simulink model "aconserversimulation"  (R2019b)
settings: Solver=FixedStepAuto  StartTime=0.0  StopTime=30  RelTol=1e-3
undefined symbols (not defined in the file or in its folder): Acid, Lead, sigbuilder_block
libraries: powerlib x39, simulink x14, powerlib_extras x9, electricdrivelib x3, re_lib x1
(part 1 of 2)
settings Model: Creator=28721  LastModifiedBy=conqu
settings SolverCC: ZeroCrossAlgorithm=Adaptive  AlgebraicLoopSolver=LineSearch
settings DataIOCC: ReturnWorkspaceOutputs=off
settings DebuggingCC: MaxConsecutiveZCsMsg=none  ArithmeticOperatorsInVariantConditions=warning
settings SFSimCC: SimUseLocalCustomCode=off  CustomCodeUndefinedFunction=UseInterfaceOnly
settings RTWCC: RTWUseLocalCustomCode=off

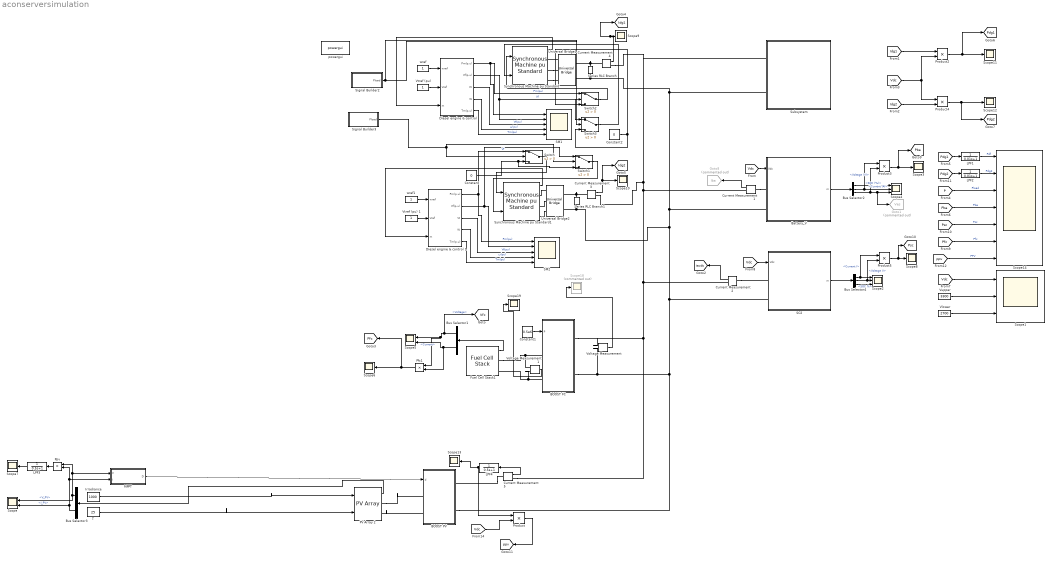
== system aconserversimulation ==
  BOOST FC : Subsystem
  BOOST PV : Subsystem
  Battery_V : Subsystem
      mask Display: image('D:\u盘文件\仿真\封装图片\timg (1).jpg');
  Bus Selector2 : BusSelector  OutputSignals=SOC (%),Current (A),Voltage (V)
  Bus Selector4 : BusSelector  OutputSignals=Current I,Voltage V,SOC %
  Bus Selector1 : BusSelector  OutputSignals=Voltage,Current
  Bus Selector3 : BusSelector  OutputSignals=V_PV,I_PV
  Constant : Constant  Value=0
  Constant1 : Constant  Value=0.5e6
  Constant2 : Constant  Value=0
  Current Measurement{1..5} (5 alike) : powerlib/Measurements/Current Measurement  PhasorSimulation=off  OutputType=Complex  PSBequivalent=0
      settings: SourceProductName=Simscape Electrical
  "Diesel engine & control " : Subsystem
  Diesel engine & control 1 : Subsystem
  Fuel Cell Stack1 : electricdrivelib/Extra Sources/Fuel Cell Stack  PresetModel=No (User-Defined)  FcType=Proton Exchange Membrane (PEM)  Detailed=Simplified  Eoc=[1600,1500]  NomVI=[800,2000]  EndVI=[1000,1800]  Nc=900  n=55  TOp=65  AirFr=2100  SuppPress=[1.5,1]  Comp=[99.95,21,1]  SignX=off  SignY=off  FlowRateH2=off  FlowRateAir=off  SystemTemp=off  SystemPH2=off  SystemPAir=off  FCDyn=on  FC_tau=1  Peak_O2=80  V_Under=10
      settings: SourceProductName=Simscape Electrical  SourceProductBaseCode=PS
  Goto1 : Goto  Commented=on  GotoTag=Ves  TagVisibility=global
  Goto8 : Goto  Commented=on  GotoTag=Iba  TagVisibility=global
  Irradiance : Constant  Value=1000
  LPF1 : TransferFcn  Denominator=[0.01 1]
  LPF2 : TransferFcn  Denominator=[0.01 1]
  LPF3 : TransferFcn  Denominator=[0.5 1]
  LPF4 : TransferFcn  Denominator=[0.5 1]
  MPPT : Subsystem
  PV Array 2 : re_lib/Solar/PV Array  Npar=100  Nser=55  PlotType=array @ 1000 W/m2 & specified temperatures  S_vec="[ 1000  500  100 ]"  Temp_C_vec="[ 50 25  ]"  ModuleName=Advanced Renewable Energy AREi-210W-M6-G  PlotWhenSelected=off  Pm=210.384  Ncell=60  Voc=36.3  Isc=7.74  Vm=29.22  Im=7.2  beta_Voc_pc=-0.35339  alpha_Isc_pc=0.055349  beta_Voc=-0.12828  alpha_Isc=0.004284  IL=7.7542  I0=2.0567e-10  nI=0.96787  Rsh=203.5777  Rs=0.37252  BAL=on  Tc=1e-6  Tfilter=5e-5
      link override Diode Rsh/Rsh_array_5%Sref: Value=Rsh_array5pc
      settings: SourceProductName=Simscape Electrical
  Pfc1 : Product
  Ppv : Product
  Product{,2..5} (5 alike) : Product
  SC2 : Subsystem
      mask Display: image('D:\u盘文件\仿真\封装图片\timg.jpg');
  SM1 : Scope  NumInputPorts=5
  SM2 : Scope  NumInputPorts=5
  Scope : Scope  NumInputPorts=2
  Scope1 : Scope  NumInputPorts=3
  Scope{3,6..13,19} (10 alike) : Scope
  Scope14 : Scope  NumInputPorts=7
  Scope18 : Scope  Commented=on
  Scope2 : Scope  NumInputPorts=3
  Scope4 : Scope  NumInputPorts=3
  Scope5 : Scope  NumInputPorts=2
  Series RLC Branch : powerlib/Elements/Series RLC Branch  LConnTagsString=__new0  RConnTagsString=__new0  BranchType=C  Resistance=1  Inductance=1e-3  SetiL0=off  InitialCurrent=0  Capacitance=1000e-6  Setx0=off  InitialVoltage=0  Measurements=None
      settings: SourceProductName=Simscape Electrical
  Series RLC Branch1 : powerlib/Elements/Series RLC Branch  LConnTagsString=__new0  RConnTagsString=__new0  BranchType=C  Resistance=1  Inductance=1e-3  SetiL0=off  InitialCurrent=0  Capacitance=1000e-6  Setx0=off  InitialVoltage=0  Measurements=None
      settings: SourceProductName=Simscape Electrical
  Signal Builder2 : Subsystem  Tag=STV Subsys  LoadFcn=sigbuilder_block('load');  StartFcn=sigbuilder_block('start');  StopFcn=sigbuilder_block('stop');  ClipboardFcn=sigbuilder_block('clipboard');  mask(Sigbuilder block){tuvar=[0:10]}
      mask help: Simulink:masks:SigbuilderBlock_MD
      mask init:
      | if ~strcmp(get_param(bdroot(gcbh),'SimulationStatus'),'stopped') tuvar = sigbuilder_block('maskInit'); end
      settings: CopyFcn=sigbuilder_block('copy');  DeleteFcn=sigbuilder_block('delete');  ModelCloseFcn=sigbuilder_block('modelClose');  PreSaveFcn=sigbuilder_block('preSave');  PauseFcn=sigbuilder_block('pause');  ContinueFcn=sigbuilder_block('continue');  NameChangeFcn=sigbuilder_block('namechange');  OpenFcn=sigbuilder_block('open',[381.6 135 550.8 400.2 ]);  CloseFcn=sigbuilder_block('close');
      mask Display: plot(0, 0, 100, 100,[2, 2, 32, 32, 2], [68, 8, 8, 68, 68],[32, 2], [38, 38], [32, 19, 2],[53, 60, 44], [32, 17, 17, 2],[16, 16, 31, 31]);txt = getActiveGroup(gcbh);text(2, 100, txt,'verticalAlignment', 'top');
  Signal Builder3 : Subsystem  Tag=STV Subsys  LoadFcn=sigbuilder_block('load');  StartFcn=sigbuilder_block('start');  StopFcn=sigbuilder_block('stop');  ClipboardFcn=sigbuilder_block('clipboard');  mask(Sigbuilder block){tuvar=[0:10]}
      mask help: Simulink:masks:SigbuilderBlock_MD
      mask init:
      | if ~strcmp(get_param(bdroot(gcbh),'SimulationStatus'),'stopped') tuvar = sigbuilder_block('maskInit'); end
      settings: CopyFcn=sigbuilder_block('copy');  DeleteFcn=sigbuilder_block('delete');  ModelCloseFcn=sigbuilder_block('modelClose');  PreSaveFcn=sigbuilder_block('preSave');  PauseFcn=sigbuilder_block('pause');  ContinueFcn=sigbuilder_block('continue');  NameChangeFcn=sigbuilder_block('namechange');  OpenFcn=sigbuilder_block('open',[381.6 135 550.8 400.2 ]);  CloseFcn=sigbuilder_block('close');
      mask Display: plot(0, 0, 100, 100,[2, 2, 32, 32, 2], [68, 8, 8, 68, 68],[32, 2], [38, 38], [32, 19, 2],[53, 60, 44], [32, 17, 17, 2],[16, 16, 31, 31]);txt = getActiveGroup(gcbh);text(2, 100, txt,'verticalAlignment', 'top');
  Subsystem : Subsystem
  Switch{,1..3} (4 alike) : Switch  Criteria=u2 > Threshold
  Synchronous Machine pu Standard : powerlib/Machines/Synchronous Machine pu Standard  PresetModel=No  MechanicalLoad=Mechanical power Pm  ShowDetailedParameters=on  RotorType=Salient-pole  Units=per unit standard parameters  MeasurementBus=off  NominalParameters="[3e6  2450 60]"  Reactances1=[ 1.81, 0.3, 0.23, 1.76, 0.65, 0.25, 0.15 ]  Reactances2=[ 1.56, 0.296, 0.177, 1.06, 0.177, 0.052 ]  dAxisTimeConstants=Short-circuit  qAxisTimeConstants=Open-circuit  TimeConstants1="[ 4.4849  0.0681  0.1  ]"  TimeConstants2=[ 8.0, 0.03, 1.0, 0.07 ]  TimeConstants3="[  4.49  0.0681  0.0513  ]"  TimeConstants4=[ 8.0, 0.03, 0.3371, 0.0295 ]  TimeConstants5=[ 3.7, 0.05, 0.05 ]  TimeConstants6=[ 1.3201, 0.023, 1.0, 0.07 ]  TimeConstants7=[ 3.7, 0.05, 0.05 ]  TimeConstants8=[ 1.3201, 0.0231, 0.3371, 0.0295 ]  StatorResistance=0.0036  Mechanical="[ 1.07  0 2]"  PolePairs=20  InitialConditions="[ 0  0  0  0  0  0  0  0  1 ]"  SetSaturation=on  Saturation=[0.6404,0.7127,0.8441,0.9214,0.9956,1.082,1.19,1.316,1.457;0.7,0.7698,0.8872,0.9466,0.9969,1.046,1.1,1.151,1.201]  LoadFlowParameters=[1,0,0,0,0]  TsPowergui=0  TsBlock=-1  IterativeModel=Trapezoidal non iterative  IterativeDiscreteModel=Trapezoidal non iterative  BusType=PV  Pref=0  Qref=0  Qmin=-inf  Qmax=inf  PLF=0  QLF=0
      settings: SourceProductName=Simscape Electrical
  Synchronous Machine pu Standard1 : powerlib/Machines/Synchronous Machine pu Standard  PresetModel=No  MechanicalLoad=Mechanical power Pm  ShowDetailedParameters=on  RotorType=Salient-pole  Units=per unit standard parameters  MeasurementBus=off  NominalParameters="[3e6  2450 60]"  Reactances1=[ 1.81, 0.3, 0.23, 1.76, 0.65, 0.25, 0.15 ]  Reactances2=[ 1.56, 0.296, 0.177, 1.06, 0.177, 0.052 ]  dAxisTimeConstants=Short-circuit  qAxisTimeConstants=Open-circuit  TimeConstants1="[ 4.4849  0.0681  0.1  ]"  TimeConstants2=[ 8.0, 0.03, 1.0, 0.07 ]  TimeConstants3="[  4.49  0.0681  0.0513  ]"  TimeConstants4=[ 8.0, 0.03, 0.3371, 0.0295 ]  TimeConstants5=[ 3.7, 0.05, 0.05 ]  TimeConstants6=[ 1.3201, 0.023, 1.0, 0.07 ]  TimeConstants7=[ 3.7, 0.05, 0.05 ]  TimeConstants8=[ 1.3201, 0.0231, 0.3371, 0.0295 ]  StatorResistance=0.0036  Mechanical="[ 1.07  0 2]"  PolePairs=20  InitialConditions="[ 0  0  0  0  0  0  0  0  1 ]"  SetSaturation=on  Saturation=[0.6404,0.7127,0.8441,0.9214,0.9956,1.082,1.19,1.316,1.457;0.7,0.7698,0.8872,0.9466,0.9969,1.046,1.1,1.151,1.201]  LoadFlowParameters=[1,0,0,0,0]  TsPowergui=0  TsBlock=-1  IterativeModel=Trapezoidal non iterative  IterativeDiscreteModel=Trapezoidal non iterative  BusType=PV  Pref=0  Qref=0  Qmin=-inf  Qmax=inf  PLF=0  QLF=0
      settings: SourceProductName=Simscape Electrical
  T : Constant  Value=25
  Universal Bridge1 : powerlib/Power Electronics/Universal Bridge  Arms=3  SnubberResistance=1e5  SnubberCapacitance=inf  Device=Diodes  Ron=1e-3  Lon=0  ForwardVoltages="[  0  0  ]"  ForwardVoltage=0  GTOparameters=[ 10e-6 , 20e-6 ]  IGBTparameters=[ 1e-6 , 2e-6 ]  Measurements=Device currents  Measurements_2=None  converterType=Rectifier
      settings: SourceProductName=Simscape Electrical
  Universal Bridge2 : powerlib/Power Electronics/Universal Bridge  Arms=3  SnubberResistance=1e5  SnubberCapacitance=inf  Device=Diodes  Ron=1e-3  Lon=0  ForwardVoltages="[  0  0  ]"  ForwardVoltage=0  GTOparameters=[ 10e-6 , 20e-6 ]  IGBTparameters=[ 1e-6 , 2e-6 ]  Measurements=Device currents  Measurements_2=None  converterType=Rectifier
      settings: SourceProductName=Simscape Electrical
  Vlower : Constant  Value=2700
  Voltage Measurement : powerlib/Measurements/Voltage Measurement  PhasorSimulation=off  OutputType=Complex  PSBequivalent=0
      settings: SourceProductName=Simscape Electrical
  Voltage Measurement1 : powerlib/Measurements/Voltage Measurement  PhasorSimulation=off  OutputType=Complex  PSBequivalent=0
      settings: SourceProductName=Simscape Electrical
  "Vtref (pu) " : Constant
  Vtref (pu) 1 : Constant
  Vupper : Constant  Value=3300
  powergui : powerlib/powergui  Priority=1  SimulationMode=Discrete  SampleTime=50e-6  frequency=60  Iterations=50  frequencyindice=0  Pbase=100e6  ErrMax=1e-4  UnitsV=kV  UnitsW=MW  buscounter=0  FunctionMessages=off  echomessages=off  EnableUseOfTLC=off  CurrentSourceSwitches=off  DisableSnubberDevices=off  DisableRonSwitches=off  DisableVfSwitches=off  DisplayEquations=off  AutomaticDiscreteSolvers=off  SolverType=Tustin/Backward Euler (TBE)  Interpol=off  ExternalGateDelay=off  methode=off  Ts=100  x0status=blocks  SPID=off  SwTol=0  HookPort=off  NonlinearTolerance=1e-4  nMaxIteration=100  ContinueOnMaxIteration=off  RestoreLinks=warning  ResistiveCurrentMeasurement=off  Frange=[0:2:500]  Ylog=off  Xlog=on  ShowGrid=off  save=off  variable=ZData  structure=Vdc  ZoomFFT=off  StartTime=0.0  cycles=1  DisplayStyle=1  fundamental=1  FreqAxis=off  MaxFrequency=1000  frequencyindicesteady=1  RmsSteady=1  display=off
      settings: SourceProductName=Simscape Electrical
  wref : Constant
  wref1 : Constant
  tag scope: Idg1=global, Idg2=global, Pba=global, Pdg1=global, Pdg2=global, Pfc=global, Psc=global, Vfc=global, iscdc=global, ppv=global
  wires:
  "Diesel engine & control "/4(W) -> SM1/4  "ω(pu)"
  "Diesel engine & control "/5(Tm(p.u)) -> SM1/5  "Tm(pu)"
  "Vtref (pu) "/1 -> "Diesel engine & control "/2(Vref)
  Synchronous Machine pu Standard/1 -> "Diesel engine & control "/3(m)
  "Diesel engine & control "/1(Pm(p.u)) -> Switch2/1, SM1/1  "Pm(pu)"
  "Diesel engine & control "/3(Vt) -> SM1/3  "Vt(pu)"
  "Diesel engine & control "/2(Vf(p.u)) -> Switch3/1, SM1/2  "Vf"
  wref/1 -> "Diesel engine & control "/1(wref)
  Bus Selector2/1 -> Scope4/1  "<SOC (%)>"
  Battery_V/1(m) -> Bus Selector2/1
  Bus Selector2/2 -> Product3/1, Scope4/2  "<Current (A)>"
  Bus Selector2/3 -> Product3/2, Goto1/1, Scope4/3  "<Voltage (V)>"
  Product3/1 -> [Pba], Scope3/1
  [Vdc] -> Battery_V/1(Vdc)
  Current Measurement4/1 -> [Idg1], Scope9/1
  [Idg1] -> Product2/1
  [Idg2] -> Product4/2
  [Vdc] -> Product2/2, Product4/1
  Product4/1 -> [Pdg2], Scope12/1
  Product2/1 -> Scope11/1, [Pdg1]
  Current Measurement1/1 -> Goto8/1
  LPF1/1 -> Scope14/1  "Pdf"
  LPF2/1 -> Scope14/2  "Pdg2"
  [P] -> Scope14/3  "Pload"
  wref1/1 -> Diesel engine & control 1/1(wref)
  Synchronous Machine pu Standard1/1 -> Diesel engine & control 1/3(m)
  Diesel engine & control 1/2(Vf(p.u)) -> Switch1/1, SM2/2  "Vf"
  Diesel engine & control 1/3(Vt) -> SM2/3  "Vt(pu)"
  Vtref (pu) 1/1 -> Diesel engine & control 1/2(Vref)
  Diesel engine & control 1/1(Pm(p.u)) -> Switch/1, SM2/1  "Pm(pu)"
  Diesel engine & control 1/5(Tm(p.u)) -> SM2/5  "Tm(pu)"
  Diesel engine & control 1/4(W) -> SM2/4  "ω(pu)"
  Current Measurement3/1 -> [Idg2], Scope10/1
  [Pba] -> Scope14/4  "Pba"
  [Vdc] -> Scope1/1
  Current Measurement2/1 -> [iscdc]
  Bus Selector4/3 -> Scope2/3  "<SOC %>"
  SC2/1(m) -> Bus Selector4/1
  [Vdc] -> SC2/1(Vdc)
  Bus Selector4/1 -> Product5/1, Scope2/1  "<Current I>"
  Product5/1 -> [Psc], Scope8/1
  Bus Selector4/2 -> Product5/2, Scope2/2  "<Voltage V>"
  [Psc] -> Scope14/5  "Psc"
  Constant1/1 -> BOOST FC/1(P)
  Bus Selector1/1 -> [Vfc], Pfc1/1, Scope5/1  "<Voltage>"
  Fuel Cell Stack1/1 -> Bus Selector1/1
  Pfc1/1 -> [Pfc], Scope6/1
  Bus Selector1/2 -> Pfc1/2, Scope5/2  "<Current>"
  [Pfc] -> Scope14/6  "Pfc"
  [Pdg2] -> LPF2/1
  [Pdg1] -> LPF1/1
  [ppv] -> Scope14/7  "PPV"
  Vupper/1 -> Scope1/2
  Vlower/1 -> Scope1/3
  Voltage Measurement/1 -> Scope18/1
  Voltage Measurement1/1 -> Scope19/1
  Constant/1 -> Switch1/3, Switch/3
  Switch/1 -> Synchronous Machine pu Standard1/1
  Switch1/1 -> Synchronous Machine pu Standard1/2
  Signal Builder3/1(Pload) -> Switch/2, Switch1/2
  Product/1 -> [ppv]
  [Vdc] -> Product/2
  Bus Selector3/2 -> Scope/2, Ppv/2, MPPT/2(I)  "<I_PV>"
  LPF4/1 -> Product/1, Scope13/1
  Irradiance/1 -> PV Array 2/1
  LPF3/1 -> Scope7/1
  Current Measurement5/1 -> LPF4/1
  MPPT/1(D) -> BOOST PV/1(d)
  Ppv/1 -> LPF3/1
  PV Array 2/1 -> Bus Selector3/1
  Bus Selector3/1 -> Scope/1, Ppv/1, MPPT/1(V)  "<V_PV>"
  T/1 -> PV Array 2/2
  Switch2/1 -> Synchronous Machine pu Standard/1
  Switch3/1 -> Synchronous Machine pu Standard/2
  Constant2/1 -> Switch2/3, Switch3/3
  Signal Builder2/1(Pload) -> Switch3/2, Switch2/2
  connections:
  Synchronous Machine pu Standard/RConn2 -- Universal Bridge1/LConn2
  Universal Bridge1/LConn1 -- Synchronous Machine pu Standard/RConn1
  Synchronous Machine pu Standard/RConn3 -- Universal Bridge1/LConn3
  Current Measurement1/LConn1 -- Battery_V/LConn1
  Voltage Measurement/LConn2 -- BOOST PV/RConn2 -- Series RLC Branch1/RConn1 -- Universal Bridge2/RConn2 -- Battery_V/LConn2 -- Series RLC Branch/RConn1 -- Universal Bridge1/RConn2 -- Subsystem/LConn2 -- SC2/LConn2 -- BOOST FC/RConn2
  Current Measurement2/RConn1 -- Current Measurement3/RConn1 -- Current Measurement4/RConn1 -- Subsystem/LConn1 -- Current Measurement1/RConn1 -- Current Measurement5/RConn1 -- Voltage Measurement/LConn1 -- BOOST FC/RConn1
  Current Measurement3/LConn1 -- Series RLC Branch1/LConn1 -- Universal Bridge2/RConn1
  Synchronous Machine pu Standard1/RConn2 -- Universal Bridge2/LConn2
  Universal Bridge2/LConn1 -- Synchronous Machine pu Standard1/RConn1
  Synchronous Machine pu Standard1/RConn3 -- Universal Bridge2/LConn3
  Current Measurement4/LConn1 -- Series RLC Branch/LConn1 -- Universal Bridge1/RConn1
  Current Measurement2/LConn1 -- SC2/LConn1
  BOOST FC/LConn2 -- Voltage Measurement1/LConn2 -- Fuel Cell Stack1/RConn2
  Fuel Cell Stack1/RConn1 -- Voltage Measurement1/LConn1 -- BOOST FC/LConn1
  Current Measurement5/LConn1 -- BOOST PV/RConn1
  PV Array 2/RConn1 -- BOOST PV/LConn1
  PV Array 2/RConn2 -- BOOST PV/LConn2

== system aconserversimulation/BOOST FC ==
  P : Inport
  Current Loop : Subsystem
  Current Measurement1 : powerlib/Measurements/Current Measurement  PhasorSimulation=off  OutputType=Complex  PSBequivalent=0
      settings: SourceProductName=Simscape Electrical
  Divide : Product  Inputs=*/
  Series RLC Branch7 : powerlib/Elements/Series RLC Branch  LConnTagsString=__new0  RConnTagsString=__new0  BranchType=C  Resistance=1  Inductance=1e-3  SetiL0=off  InitialCurrent=0  Capacitance=2000e-6  Setx0=off  InitialVoltage=0  Measurements=None
      settings: SourceProductName=Simscape Electrical
  boost converter : Subsystem
  Vdc+ : PMIOPort  Side=Right
  V+ : PMIOPort  Port=2  Side=Left
  Vdc- : PMIOPort  Port=3  Side=Right
  V- : PMIOPort  Port=4  Side=Left
  wires:
  Current Loop/1(d) -> boost converter/1(duty cycle)
  Current Measurement1/1 -> Current Loop/2(iLmes)
  Divide/1 -> Current Loop/1(iLref)
  P/1 -> Divide/1
  [Vfc] -> Divide/2
  connections:
  V+/RConn1 -- Current Measurement1/LConn1
  Current Measurement1/RConn1 -- boost converter/LConn1
  boost converter/LConn2 -- V-/RConn1
  boost converter/RConn1 -- Vdc+/RConn1 -- Series RLC Branch7/LConn1
  boost converter/RConn2 -- Vdc-/RConn1 -- Series RLC Branch7/RConn1

== system aconserversimulation/BOOST PV ==
  d : Inport
  Current Measurement2 : powerlib/Measurements/Current Measurement  PhasorSimulation=off  OutputType=Complex  PSBequivalent=0
      settings: SourceProductName=Simscape Electrical
  Current PI1 : Subsystem
  Scope4 : Scope
  boost converter : Subsystem
  Vdc+ : PMIOPort  Side=Right
  V+ : PMIOPort  Port=2  Side=Left
  Vdc- : PMIOPort  Port=3  Side=Right
  V- : PMIOPort  Port=4  Side=Left
  wires:
  d/1 -> Scope4/1, boost converter/1(duty cycle)
  connections:
  boost converter/RConn1 -- Vdc+/RConn1
  boost converter/LConn2 -- V-/RConn1
  boost converter/RConn2 -- Vdc-/RConn1
  boost converter/LConn1 -- V+/RConn1

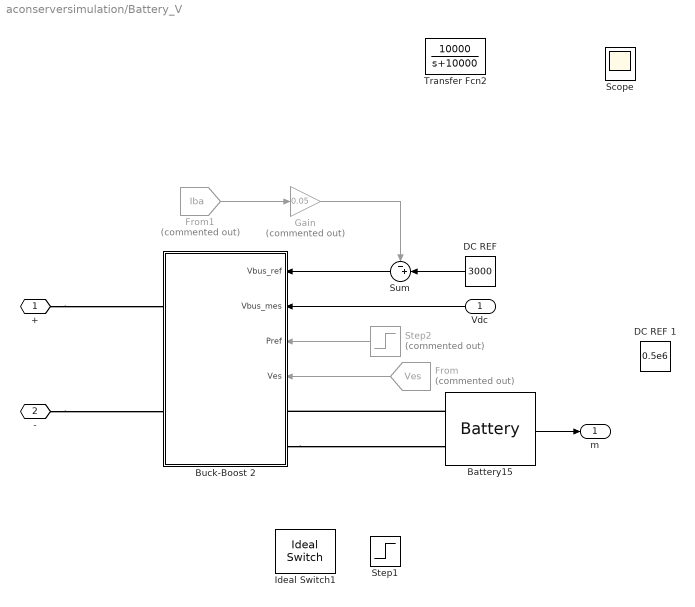
== system aconserversimulation/Battery_V ==
  Vdc : Inport
  Battery15 : electricdrivelib/Extra Sources/Battery  BatType=Lead-Acid  ShowTempParam=off  ThermalPreset=no  ShowAgeParam=off  NomV=2400  NomQ=100  SOC=40  Batt_Tr=30  PresetModel=on  MaxQ=104.1667  MinV=1800  FullV=2613.1579  Dis_rate=20  R=0.24  Normal_OP=31.0278  expZone="[2443.4211     0.33333333]"  current=[6.5 13 32.5]  Units=Time  Tci=20  NomT=20  T2=-30  MaxQ2=4.8  FullV2=7.1  Normal_OP2=5.655  expZone2="[6.58           1]"  Rca=0.6  ti=2000  Dp=0  Neq0=0  Tsim=1e6  Ta1=25  Qeol=5.4*0.9  Reol=0.013333*1.2  Char_age=[2.3478, 3]  Dis_age=[2.3478, 10]  N1=1500  N2=10500  N3=1000  N4=1400  Ta2=45  N5=950
      settings: SourceProductName=Simscape Electrical
  Buck-Boost 2 : Subsystem
  "DC REF " : Constant  Value=3000
  DC REF 1 : Constant  Value=0.5e6
  From : From  Commented=on  GotoTag=Ves  TagVisibility=global
  From1 : From  Commented=on  GotoTag=Iba  TagVisibility=global
  Gain : Gain  Commented=on  Gain=0.05
  Ideal Switch1 : powerlib/Power Electronics/Ideal Switch  Ron=0.001  Lon=0  IC=0  Rs=1e5  Cs=inf  Measurements=off
      settings: SourceProductName=Simscape Electrical
  Scope : Scope  NumInputPorts=2
  Step1 : Step  Time=2  SampleTime=0
  Step2 : Step  Commented=on  Time=3  Before=0.5e6  After=0.8e6  SampleTime=0
  Sum : Sum  Inputs=-+|
  Transfer Fcn2 : TransferFcn  Numerator=[10000]  Denominator=[1 10000]
  + : PMIOPort  Side=Left
  - : PMIOPort  Port=2  Side=Left
  m : Outport  VectorParamsAs1DForOutWhenUnconnected=off
  wires:
  Battery15/1 -> m/1
  Vdc/1 -> Buck-Boost 2/2(Vbus_mes)
  "DC REF "/1 -> Sum/2
  Sum/1 -> Buck-Boost 2/1(Vbus_ref)
  From1/1 -> Gain/1
  Gain/1 -> Sum/1
  From/1 -> Buck-Boost 2/4(Ves)
  Step2/1 -> Buck-Boost 2/3(Pref)
  connections:
  -/RConn1 -- Buck-Boost 2/RConn2
  Buck-Boost 2/LConn2 -- Battery15/LConn2
  +/RConn1 -- Buck-Boost 2/RConn1
  Battery15/LConn1 -- Buck-Boost 2/LConn1

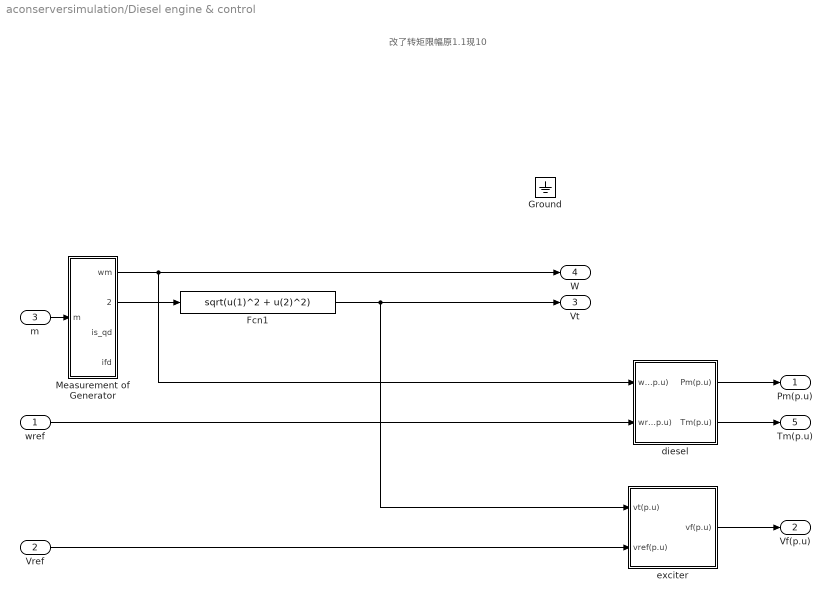
== system aconserversimulation/Diesel engine & control  ==
  note: 改了转矩限幅原1.1现10
  wref : Inport
  Vref : Inport  Port=2
  m : Inport  Port=3
  Fcn1 : Fcn  Expr=sqrt(u(1)^2 + u(2)^2)
  Ground : Ground
  Measurement of Generator : Subsystem
  diesel : Subsystem
  exciter : Subsystem
  Pm(p.u) : Outport  VectorParamsAs1DForOutWhenUnconnected=off
  Vf(p.u) : Outport  Port=2  VectorParamsAs1DForOutWhenUnconnected=off
  Vt : Outport  Port=3  VectorParamsAs1DForOutWhenUnconnected=off
  W : Outport  Port=4  VectorParamsAs1DForOutWhenUnconnected=off
  Tm(p.u) : Outport  Port=5  VectorParamsAs1DForOutWhenUnconnected=off
  wires:
  m/1 -> Measurement of Generator/1(m)
  Measurement of Generator/2(vs_qd) -> Fcn1/1
  Fcn1/1 -> exciter/1(vt(p.u)), Vt/1
  Measurement of Generator/1(wm) -> diesel/1(wm(p.u)), W/1
  wref/1 -> diesel/2(wref(p.u))
  diesel/2(Tm(p.u)) -> Tm(p.u)/1
  diesel/1(Pm(p.u)) -> Pm(p.u)/1
  Vref/1 -> exciter/2(vref(p.u))
  exciter/1(vf(p.u)) -> Vf(p.u)/1

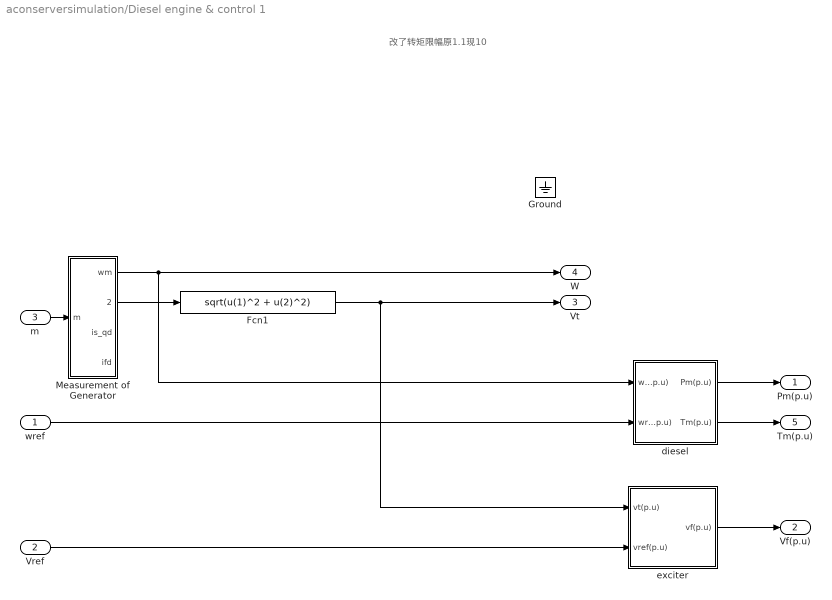
== system aconserversimulation/Diesel engine & control 1 ==
  note: 改了转矩限幅原1.1现10
  wref : Inport
  Vref : Inport  Port=2
  m : Inport  Port=3
  Fcn1 : Fcn  Expr=sqrt(u(1)^2 + u(2)^2)
  Ground : Ground
  Measurement of Generator : Subsystem
  diesel : Subsystem
  exciter : Subsystem
  Pm(p.u) : Outport  VectorParamsAs1DForOutWhenUnconnected=off
  Vf(p.u) : Outport  Port=2  VectorParamsAs1DForOutWhenUnconnected=off
  Vt : Outport  Port=3  VectorParamsAs1DForOutWhenUnconnected=off
  W : Outport  Port=4  VectorParamsAs1DForOutWhenUnconnected=off
  Tm(p.u) : Outport  Port=5  VectorParamsAs1DForOutWhenUnconnected=off
  wires:
  m/1 -> Measurement of Generator/1(m)
  Measurement of Generator/2(vs_qd) -> Fcn1/1
  Fcn1/1 -> exciter/1(vt(p.u)), Vt/1
  Measurement of Generator/1(wm) -> diesel/1(wm(p.u)), W/1
  wref/1 -> diesel/2(wref(p.u))
  diesel/2(Tm(p.u)) -> Tm(p.u)/1
  diesel/1(Pm(p.u)) -> Pm(p.u)/1
  Vref/1 -> exciter/2(vref(p.u))
  exciter/1(vf(p.u)) -> Vf(p.u)/1

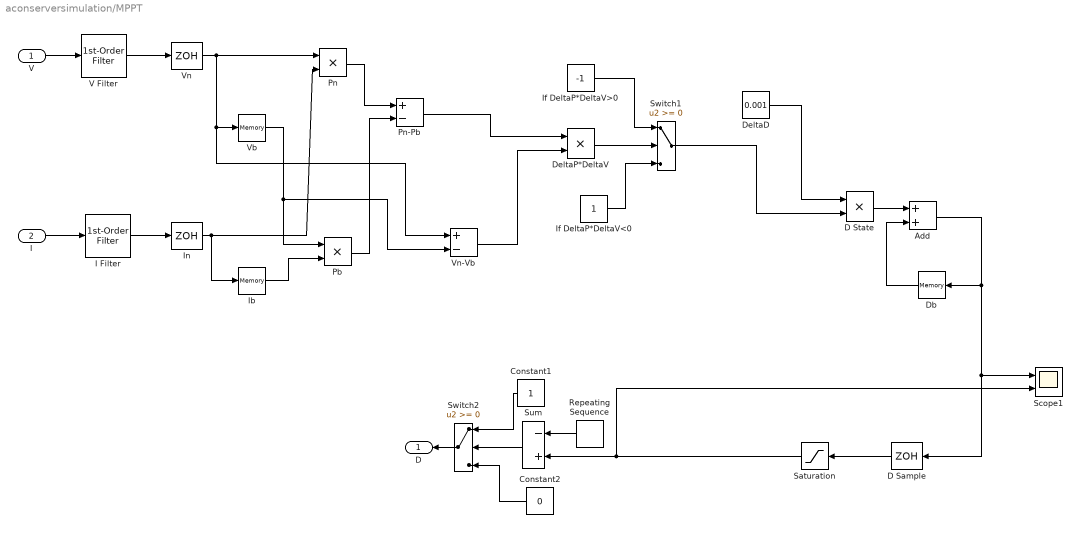
== system aconserversimulation/MPPT ==
  V : Inport
  I : Inport  Port=2
  Add : Sum
  Constant1 : Constant  SampleTime=-1
  Constant2 : Constant  Value=0  SampleTime=-1
  D Sample : ZeroOrderHold  SampleTime=1e-4
  D State : Product  RndMeth=Zero
  Db : Memory  InheritSampleTime=on  LinearizeAsDelay=on
  DeltaD : Constant  Value=0.001
  DeltaP*DeltaV : Product  RndMeth=Zero
  I Filter : powerlib_extras/Control  Blocks/1st-Order  Filter  FilterType=Lowpass  Tc=1e-3  Initialize=off  Vac_Init=[0.8 -25 60]  Vdc_Init=-0.4  PlotResponse=off  param1=[1 500 1]
      settings: SourceProductName=Simscape Electrical  SourceProductBaseCode=PS
  Ib : Memory  InheritSampleTime=on  LinearizeAsDelay=on
  If DeltaP*DeltaV<0 : Constant
  If DeltaP*DeltaV>0 : Constant  Value=-1
  In : ZeroOrderHold  SampleTime=1e-4
  Pb : Product  RndMeth=Zero
  Pn : Product  RndMeth=Zero
  Pn-Pb : Sum  Inputs=+-
  Repeating Sequence : simulink/Sources/Repeating Sequence  rep_seq_t=[0 3.9e-3 4e-3]  rep_seq_y=[0 1 0]
  Saturation : Saturate  UpperLimit=0.8  LowerLimit=0
  Scope1 : Scope  NumInputPorts=2
  Sum : Sum  Inputs=-+  SaturateOnIntegerOverflow=on
  Switch1 : Switch
  Switch2 : Switch
  V Filter : powerlib_extras/Control  Blocks/1st-Order  Filter  FilterType=Lowpass  Tc=1e-3  Initialize=off  Vac_Init=[0.8 -25 60]  Vdc_Init=-0.4  PlotResponse=off  param1=[1 500 1]
      settings: SourceProductName=Simscape Electrical  SourceProductBaseCode=PS
  Vb : Memory  InheritSampleTime=on  LinearizeAsDelay=on
  Vn : ZeroOrderHold  SampleTime=1e-4
  Vn-Vb : Sum  Inputs=+-
  D : Outport  VectorParamsAs1DForOutWhenUnconnected=off
  wires:
  V/1 -> V Filter/1
  I/1 -> I Filter/1
  V Filter/1 -> Vn/1
  I Filter/1 -> In/1
  In/1 -> Ib/1, Pn/2
  Vn/1 -> Pn/1, Vb/1, Vn-Vb/1
  Ib/1 -> Pb/2
  Vb/1 -> Pb/1, Vn-Vb/2
  Pn/1 -> Pn-Pb/1
  Pb/1 -> Pn-Pb/2
  D State/1 -> Add/1
  Constant2/1 -> Switch2/3
  Constant1/1 -> Switch2/1
  Sum/1 -> Switch2/2
  Repeating Sequence/1 -> Sum/1
  Add/1 -> Db/1, D Sample/1, Scope1/1
  Switch2/1 -> D/1
  Db/1 -> Add/2
  D Sample/1 -> Saturation/1
  Pn-Pb/1 -> DeltaP*DeltaV/1
  Vn-Vb/1 -> DeltaP*DeltaV/2
  DeltaP*DeltaV/1 -> Switch1/2
  If DeltaP*DeltaV>0/1 -> Switch1/1
  If DeltaP*DeltaV<0/1 -> Switch1/3
  Switch1/1 -> D State/2
  DeltaD/1 -> D State/1
  Saturation/1 -> Sum/2, Scope1/2

== system aconserversimulation/SC2 ==
  Vdc : Inport
  "Buck-Boost 1 " : Subsystem
  DC REF 1 : Constant  Value=3000
  Gain : Gain  Gain=0.1
  Sum : Sum  Inputs=-+|
  Supercapacitor : electricdrivelib/Extra Sources/Supercapacitor  C=2200  Rdc=8.9e-3  Voltage=1500  Ns=18  Np=1  Vinit=1200  Temp=25  PresetModel=off  EstParam=off  Nc=1  r=1e-9  epsilon=6.0208e-10  Ich=10  Vstern="[0.161  2.7  7.8]"  Self_dis=on  Ioc=10  Vself="[48  47.8  47.06  44.65]"  demandeplot=off  I="[10  20 100  500]"  Units=sec  Vmax=0  If=0  deltaV=0  alpha=0  sec=0
      settings: SourceProductName=Simscape Electrical  SourceProductBaseCode=PS
  Transfer Fcn2 : TransferFcn  Numerator=[1 0]  Denominator=[1 1000]
  + : PMIOPort  Side=Left
  - : PMIOPort  Port=2  Side=Left
  m : Outport  VectorParamsAs1DForOutWhenUnconnected=off
  wires:
  Supercapacitor/1 -> m/1
  Vdc/1 -> "Buck-Boost 1 "/2(Vbus_mes)
  [iscdc] -> Gain/1
  DC REF 1/1 -> Sum/2
  Sum/1 -> "Buck-Boost 1 "/1(Vbus_ref)
  connections:
  Supercapacitor/LConn1 -- "Buck-Boost 1 "/LConn1
  Supercapacitor/LConn2 -- "Buck-Boost 1 "/LConn2
  "Buck-Boost 1 "/RConn1 -- +/RConn1
  "Buck-Boost 1 "/RConn2 -- -/RConn1

== system aconserversimulation/Signal Builder2 ==
  Demux : Demux  Tag=STV Demux  Outputs=1
  FromWs : FromWorkspace  Tag=STV FromWs  VariableName=tuvar  SampleTime=0
      SigBuilderData=|
      | common.afterFinalStr = 'Extrapolate'
      | common.sampleTime = 0
      | dataSet.timeRange = [0 20]
      | dataSet.name = 'Group 1'
      | sbobj.Groups.Name = 'Group 1'
      | sbobj.Groups.Signals.Name = 'Pload'
      | sbobj.Groups.Signals.XData = [0 4 10 10 12 16 20]
      | sbobj.Groups.Signals.YData = [0 0 0 1 1 1 1]
      | sbobj.Groups.TimeRange = [0 20]
  Pload : Outport  Tag=STV Outport  VectorParamsAs1DForOutWhenUnconnected=off
  wires:
  FromWs/1 -> Demux/1
  Demux/1 -> Pload/1

== system aconserversimulation/Signal Builder3 ==
  Demux : Demux  Tag=STV Demux  Outputs=1
  FromWs : FromWorkspace  Tag=STV FromWs  VariableName=tuvar  SampleTime=0
      SigBuilderData=|
      | common.afterFinalStr = 'Extrapolate'
      | common.sampleTime = 0
      | dataSet.timeRange = [0 30]
      | dataSet.name = 'Group 1'
      | sbobj.Groups.Name = 'Group 1'
      | sbobj.Groups.Signals.Name = 'Pload'
      | sbobj.Groups.Signals.XData = [0 4 16 16 22 22 26 26 30]
      | sbobj.Groups.Signals.YData = [0 0 0 1 1 0 0 1 1]
      | sbobj.Groups.TimeRange = [0 30]
  Pload : Outport  Tag=STV Outport  VectorParamsAs1DForOutWhenUnconnected=off
  wires:
  FromWs/1 -> Demux/1
  Demux/1 -> Pload/1

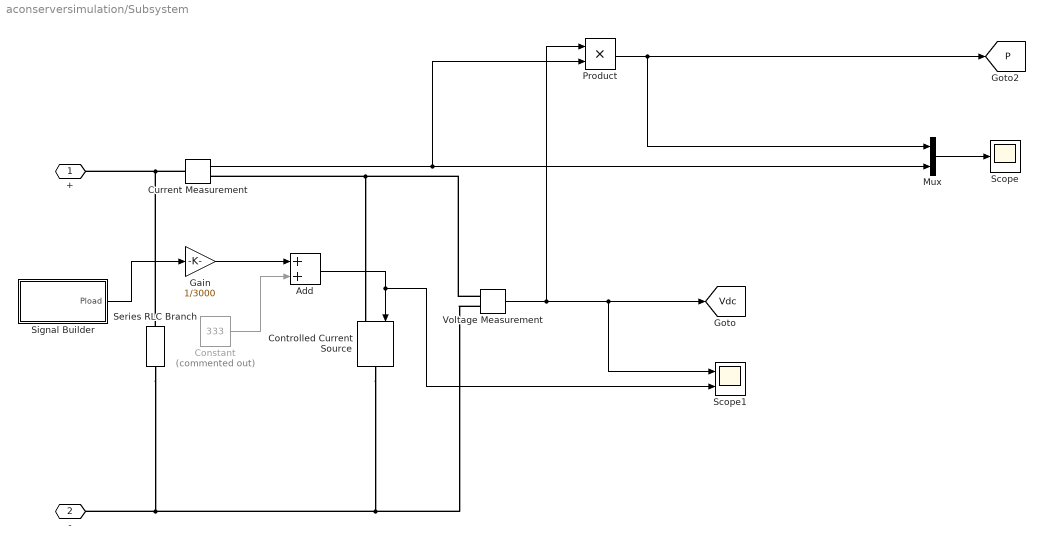
== system aconserversimulation/Subsystem ==
  Add : Sum
  Constant : Constant  Commented=on  Value=333
  Controlled Current Source : powerlib/Electrical Sources/Controlled Current Source  Initialize=on  Source_Type=AC  Amplitude=0  Phase=0  Frequency=0  Measurements=None
      settings: SourceProductName=Simscape Electrical
  Current Measurement : powerlib/Measurements/Current Measurement  PhasorSimulation=off  OutputType=Complex  PSBequivalent=0
      settings: SourceProductName=Simscape Electrical
  Gain : Gain  Gain=1/3000
  Mux : Mux  Inputs=2
  Product : Product
  Scope : Scope
  Scope1 : Scope  NumInputPorts=2
  Series RLC Branch : powerlib/Elements/Series RLC Branch  LConnTagsString=__new0  RConnTagsString=__new0  BranchType=C  Resistance=1  Inductance=1e-3  SetiL0=off  InitialCurrent=0  Capacitance=0.1  Setx0=off  InitialVoltage=1500  Measurements=None
      settings: SourceProductName=Simscape Electrical
  Signal Builder : Subsystem  Tag=STV Subsys  LoadFcn=sigbuilder_block('load');  StartFcn=sigbuilder_block('start');  StopFcn=sigbuilder_block('stop');  ClipboardFcn=sigbuilder_block('clipboard');  mask(Sigbuilder block){tuvar=[0:10]}
      mask help: Simulink:masks:SigbuilderBlock_MD
      mask init:
      | if ~strcmp(get_param(bdroot(gcbh),'SimulationStatus'),'stopped') tuvar = sigbuilder_block('maskInit'); end
      settings: CopyFcn=sigbuilder_block('copy');  DeleteFcn=sigbuilder_block('delete');  ModelCloseFcn=sigbuilder_block('modelClose');  PreSaveFcn=sigbuilder_block('preSave');  PauseFcn=sigbuilder_block('pause');  ContinueFcn=sigbuilder_block('continue');  NameChangeFcn=sigbuilder_block('namechange');  OpenFcn=sigbuilder_block('open',[381.6 135 550.8 400.2 ]);  CloseFcn=sigbuilder_block('close');
      mask Display: plot(0, 0, 100, 100,[2, 2, 32, 32, 2], [68, 8, 8, 68, 68],[32, 2], [38, 38], [32, 19, 2],[53, 60, 44], [32, 17, 17, 2],[16, 16, 31, 31]);txt = getActiveGroup(gcbh);text(2, 100, txt,'verticalAlignment', 'top');
  Voltage Measurement : powerlib/Measurements/Voltage Measurement  PhasorSimulation=off  OutputType=Complex  PSBequivalent=0
      settings: SourceProductName=Simscape Electrical
  + : PMIOPort  Side=Left
  - : PMIOPort  Port=2  Side=Left
  tag scope: P=global, Vdc=global
  wires:
  Mux/1 -> Scope/1
  Current Measurement/1 -> Mux/2, Product/2
  Product/1 -> [P], Mux/1
  Voltage Measurement/1 -> Scope1/1, [Vdc], Product/1
  Signal Builder/1(Pload) -> Gain/1
  Add/1 -> Scope1/2, Controlled Current Source/1
  Constant/1 -> Add/2
  Gain/1 -> Add/1
  connections:
  Voltage Measurement/LConn1 -- Controlled Current Source/LConn1 -- Current Measurement/RConn1
  Controlled Current Source/RConn1 -- Series RLC Branch/RConn1 -- -/RConn1 -- Voltage Measurement/LConn2
  Current Measurement/LConn1 -- Series RLC Branch/LConn1 -- +/RConn1

== system aconserversimulation/BOOST FC/Current Loop ==
  iLref : Inport
  iLmes : Inport  Port=2
  PID Controller : simulink/Continuous/PID Controller  Controller=PI  Form=Ideal  TimeDomain=Discrete-time  SampleTime=5e-6  IntegratorMethod=Forward Euler  FilterMethod=Forward Euler  ControllerParametersSource=internal  P=0.0045  I=0.20  D=0  UseFilter=on  N=100  TunerSelectOption=Transfer Function Based (PID Tuner App)  InitialConditionSource=internal  InitialConditionForIntegrator=0  InitialConditionForFilter=0  DifferentiatorICPrevScaledInput=0  ExternalReset=none  TrackingMode=off  Kt=1  LimitOutput=off  UpperSaturationLimit=inf  LowerSaturationLimit=-inf  LinearizeAsGain=on  AntiWindupMode=none  Kb=1  POutMin=[]  POutMax=[]  IOutMin=[]  IOutMax=[]  DOutMin=[]  DOutMax=[]  NOutMin=[]  NOutMax=[]  SumOutMin=[]  SumOutMax=[]  SaturationOutMin=[]  SaturationOutMax=[]  PParamMin=[]  PParamMax=[]  IParamMin=[]  IParamMax=[]  DParamMin=[]  DParamMax=[]  NParamMin=[]  NParamMax=[]  KbParamMin=[]  KbParamMax=[]  KtParamMin=[]  KtParamMax=[]  KbOutMin=[]  KbOutMax=[]  KtOutMin=[]  KtOutMax=[]  IntegratorOutMin=[]  IntegratorOutMax=[]  FilterOutMin=[]  FilterOutMax=[]  SumI1OutMin=[]  SumI1OutMax=[]  SumI2OutMin=[]  SumI2OutMax=[]  SumI3OutMin=[]  SumI3OutMax=[]  SumI4OutMin=[]  SumI4OutMax=[]  SumDOutMin=[]  SumDOutMax=[]  DifferentiatorOutMin=[]  DifferentiatorOutMax=[]  FilterDiffOutCoefMin=[]  FilterDiffOutCoefMax=[]  ReciprocalOutMin=[]  ReciprocalOutMax=[]  SumDenOutMin=[]  SumDenOutMax=[]  SumNumOutMin=[]  SumNumOutMax=[]  DivideOutMin=[]  DivideOutMax=[]  IntegratorContinuousStateAttributes=''  IntegratorStateMustResolveToSignalObject=off  IntegratorRTWStateStorageClass=Auto  FilterContinuousStateAttributes=''  FilterStateMustResolveToSignalObject=off  FilterRTWStateStorageClass=Auto  ParallelPVariant=Passthrough  IdealPVariant=InternalParameters  IVariant=InternalParameters  DVariant=Disabled  IntegratorVariant=Discrete  SatVariant=Disabled  AWVariant=Passthrough  PCopyVariant=Disabled  TRVariant=Disabled  FdbkBlocksVariant=Forward  IdealPFdbkVariant=Disabled  SatFdbkVariant=Disabled  DerivativeFilterVariant=Disabled  NVariant=Disabled  NCopyVariant=Disabled_SignalSpec  FilterICVariant=Disabled  IntegratorICVariant=InternalICs  ExternalResetVariant=Disabled  TRSumVariant=Passthrough  SumFdbkVariant=Disabled  SumVariant=Sum_PI
  Subtract : Sum  Inputs=+-
  d : Outport  VectorParamsAs1DForOutWhenUnconnected=off
  wires:
  iLmes/1 -> Subtract/2
  iLref/1 -> Subtract/1
  Subtract/1 -> PID Controller/1
  PID Controller/1 -> d/1

== system aconserversimulation/BOOST FC/boost converter ==
  duty cycle : Inport
  Diode : powerlib/Power Electronics/Diode  Ron=0.001  Lon=0  Vf=0.8  IC=0  UseSnubber=off  Rs=500  Cs=250e-9  Measurements=on
      settings: SourceProductName=Simscape Electrical
  L : powerlib/Elements/Series RLC Branch  LConnTagsString=__new0  RConnTagsString=__new0  BranchType=L  Resistance=1  Inductance=90e-3  SetiL0=off  InitialCurrent=0  Capacitance=1e-6  Setx0=off  InitialVoltage=0  Measurements=Branch current
      settings: SourceProductName=Simscape Electrical
  Mosfet : powerlib/Power Electronics/Mosfet  Ron=0.1  Lon=0  Rd=0.01  Vfd=0  IC=0  Rs=1e5  Cs=inf  Measurements=on
      settings: SourceProductName=Simscape Electrical
  Relational Operator : RelationalOperator  OutDataTypeStr=boolean  RndMeth=Nearest
  Repeating Sequence1 : simulink/Sources/Repeating Sequence  rep_seq_t=[0 5e-4 1e-3]  rep_seq_y=[0 1 0]
  Scope1 : Scope
  Vin+ : PMIOPort  Side=Left
  Vin- : PMIOPort  Port=2  Side=Left
  Vdc+ : PMIOPort  Port=3  Side=Right
  Vdc- : PMIOPort  Port=4  Side=Right
  wires:
  Repeating Sequence1/1 -> Scope1/1, Relational Operator/2
  duty cycle/1 -> Relational Operator/1
  Relational Operator/1 -> Mosfet/1
  connections:
  Vdc+/RConn1 -- Diode/RConn1
  Vin+/RConn1 -- L/LConn1
  Mosfet/RConn1 -- Vin-/RConn1 -- Vdc-/RConn1
  Mosfet/LConn1 -- L/RConn1 -- Diode/LConn1

== system aconserversimulation/BOOST PV/Current PI1 ==
  iPVref : Inport
  iPVmes : Inport  Port=2
  PID Controller : simulink/Continuous/PID Controller  Controller=PI  Form=Ideal  TimeDomain=Continuous-time  SampleTime=-1  IntegratorMethod=Forward Euler  FilterMethod=Forward Euler  ControllerParametersSource=internal  P=0.28  I=40  D=0  UseFilter=on  N=100  TunerSelectOption=Transfer Function Based (PID Tuner App)  InitialConditionSource=internal  InitialConditionForIntegrator=0  InitialConditionForFilter=0  DifferentiatorICPrevScaledInput=0  ExternalReset=none  TrackingMode=off  Kt=1  LimitOutput=off  UpperSaturationLimit=inf  LowerSaturationLimit=-inf  LinearizeAsGain=on  AntiWindupMode=none  Kb=1  POutMin=[]  POutMax=[]  IOutMin=[]  IOutMax=[]  DOutMin=[]  DOutMax=[]  NOutMin=[]  NOutMax=[]  SumOutMin=[]  SumOutMax=[]  SaturationOutMin=[]  SaturationOutMax=[]  PParamMin=[]  PParamMax=[]  IParamMin=[]  IParamMax=[]  DParamMin=[]  DParamMax=[]  NParamMin=[]  NParamMax=[]  KbParamMin=[]  KbParamMax=[]  KtParamMin=[]  KtParamMax=[]  KbOutMin=[]  KbOutMax=[]  KtOutMin=[]  KtOutMax=[]  IntegratorOutMin=[]  IntegratorOutMax=[]  FilterOutMin=[]  FilterOutMax=[]  SumI1OutMin=[]  SumI1OutMax=[]  SumI2OutMin=[]  SumI2OutMax=[]  SumI3OutMin=[]  SumI3OutMax=[]  SumI4OutMin=[]  SumI4OutMax=[]  SumDOutMin=[]  SumDOutMax=[]  DifferentiatorOutMin=[]  DifferentiatorOutMax=[]  FilterDiffOutCoefMin=[]  FilterDiffOutCoefMax=[]  ReciprocalOutMin=[]  ReciprocalOutMax=[]  SumDenOutMin=[]  SumDenOutMax=[]  SumNumOutMin=[]  SumNumOutMax=[]  DivideOutMin=[]  DivideOutMax=[]  IntegratorContinuousStateAttributes=''  IntegratorStateMustResolveToSignalObject=off  IntegratorRTWStateStorageClass=Auto  FilterContinuousStateAttributes=''  FilterStateMustResolveToSignalObject=off  FilterRTWStateStorageClass=Auto  ParallelPVariant=Passthrough  IdealPVariant=InternalParameters  IVariant=InternalParameters  DVariant=Disabled  IntegratorVariant=Continuous  SatVariant=Disabled  AWVariant=Passthrough  PCopyVariant=Disabled  TRVariant=Disabled  FdbkBlocksVariant=Forward  IdealPFdbkVariant=Disabled  SatFdbkVariant=Disabled  DerivativeFilterVariant=Disabled  NVariant=Disabled  NCopyVariant=Disabled_SignalSpec  FilterICVariant=Disabled  IntegratorICVariant=InternalICs  ExternalResetVariant=Disabled  TRSumVariant=Passthrough  SumFdbkVariant=Disabled  SumVariant=Sum_PI
  Subtract : Sum  Inputs=+-
  d : Outport  VectorParamsAs1DForOutWhenUnconnected=off
  wires:
  PID Controller/1 -> d/1
  Subtract/1 -> PID Controller/1
  iPVref/1 -> Subtract/1
  iPVmes/1 -> Subtract/2

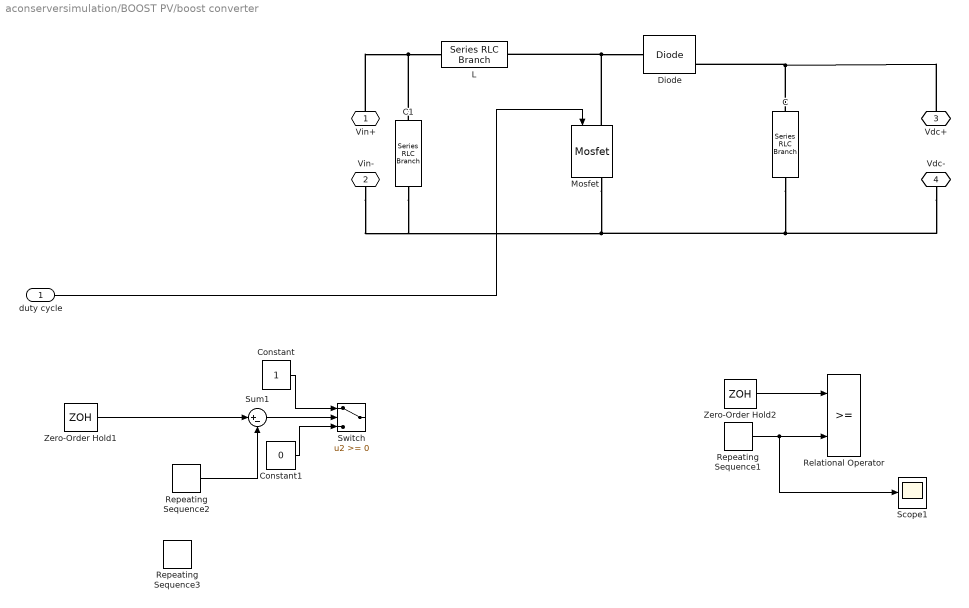
== system aconserversimulation/BOOST PV/boost converter ==
  duty cycle : Inport
  C : powerlib/Elements/Series RLC Branch  LConnTagsString=__new0  RConnTagsString=__new0  BranchType=C  Resistance=1  Inductance=1e-3  SetiL0=off  InitialCurrent=0  Capacitance=1e-3  Setx0=off  InitialVoltage=60  Measurements=None
      settings: SourceProductName=Simscape Electrical
  C1 : powerlib/Elements/Series RLC Branch  LConnTagsString=__new0  RConnTagsString=__new0  BranchType=C  Resistance=1  Inductance=1e-3  SetiL0=off  InitialCurrent=0  Capacitance=1e-3  Setx0=off  InitialVoltage=60  Measurements=None
      settings: SourceProductName=Simscape Electrical
  Constant : Constant
  Constant1 : Constant  Value=0
  Diode : powerlib/Power Electronics/Diode  Ron=0.001  Lon=0  Vf=0.8  IC=0  UseSnubber=off  Rs=500  Cs=250e-9  Measurements=on
      settings: SourceProductName=Simscape Electrical
  L : powerlib/Elements/Series RLC Branch  LConnTagsString=__new0  RConnTagsString=__new0  BranchType=L  Resistance=1  Inductance=10e-3  SetiL0=off  InitialCurrent=0  Capacitance=1e-6  Setx0=off  InitialVoltage=0  Measurements=Branch current
      settings: SourceProductName=Simscape Electrical
  Mosfet : powerlib/Power Electronics/Mosfet  Ron=0.1  Lon=0  Rd=0.01  Vfd=0  IC=0  Rs=1e5  Cs=inf  Measurements=on
      settings: SourceProductName=Simscape Electrical
  Relational Operator : RelationalOperator  OutDataTypeStr=boolean  RndMeth=Nearest
  Repeating Sequence1 : simulink/Sources/Repeating Sequence  rep_seq_t=[0 0.00005 0.0001]  rep_seq_y=[0 1 0]
  Repeating Sequence2 : simulink/Sources/Repeating Sequence  rep_seq_t=[0 0.00005 0.0001]  rep_seq_y=[0 1 0]
  Repeating Sequence3 : simulink/Sources/Repeating Sequence  rep_seq_t=[0 50e-6]  rep_seq_y=[-1 1]
  Scope1 : Scope
  Sum1 : Sum  Inputs=|+-
  Switch : Switch
  Zero-Order Hold1 : ZeroOrderHold  SampleTime=40e-5
  Zero-Order Hold2 : ZeroOrderHold  SampleTime=40e-5
  Vin+ : PMIOPort  Side=Left
  Vin- : PMIOPort  Port=2  Side=Left
  Vdc+ : PMIOPort  Port=3  Side=Right
  Vdc- : PMIOPort  Port=4  Side=Right
  wires:
  Repeating Sequence1/1 -> Scope1/1, Relational Operator/2
  Zero-Order Hold2/1 -> Relational Operator/1
  Zero-Order Hold1/1 -> Sum1/1
  Repeating Sequence2/1 -> Sum1/2
  Constant/1 -> Switch/1
  Constant1/1 -> Switch/3
  Sum1/1 -> Switch/2
  duty cycle/1 -> Mosfet/1
  connections:
  Vdc+/RConn1 -- C/LConn1 -- Diode/RConn1
  Vin+/RConn1 -- C1/LConn1 -- L/LConn1
  Vdc-/RConn1 -- C/RConn1 -- C1/RConn1 -- Vin-/RConn1 -- Mosfet/RConn1
  Mosfet/LConn1 -- Diode/LConn1 -- L/RConn1

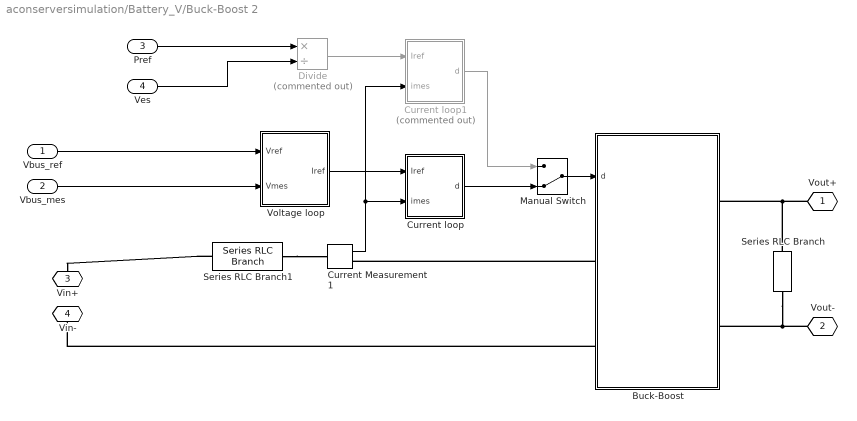
== system aconserversimulation/Battery_V/Buck-Boost 2 ==
  Vbus_ref : Inport
  Vbus_mes : Inport  Port=2
  Pref : Inport  Port=3
  Ves : Inport  Port=4
  Buck-Boost : Subsystem
  Current Measurement1 : powerlib/Measurements/Current Measurement  PhasorSimulation=off  OutputType=Complex  PSBequivalent=0
      settings: SourceProductName=Simscape Electrical
  Current loop : Subsystem
  Current loop1 : Subsystem  Commented=on
  Divide : Product  Commented=on  Inputs=*/
  Manual Switch : ManualSwitch  CurrentSetting=0
  Series RLC Branch : powerlib/Elements/Series RLC Branch  LConnTagsString=__new0  RConnTagsString=__new0  BranchType=C  Resistance=1  Inductance=1e-3  SetiL0=off  InitialCurrent=0  Capacitance=1200e-6  Setx0=off  InitialVoltage=0  Measurements=None
      settings: SourceProductName=Simscape Electrical
  Series RLC Branch1 : powerlib/Elements/Series RLC Branch  LConnTagsString=__new0  RConnTagsString=__new0  BranchType=L  Resistance=1  Inductance=9e-3  SetiL0=off  InitialCurrent=0  Capacitance=1e-6  Setx0=off  InitialVoltage=0  Measurements=None
      settings: SourceProductName=Simscape Electrical
  Voltage loop : Subsystem
  Vout+ : PMIOPort  Tag=PMCPort  Side=Right
  Vout- : PMIOPort  Tag=PMCPort  Port=2  Side=Right
  Vin+ : PMIOPort  Port=3  Side=Left
  Vin- : PMIOPort  Port=4  Side=Left
  wires:
  Vbus_ref/1 -> Voltage loop/1(Vref)
  Vbus_mes/1 -> Voltage loop/2(Vmes)
  Voltage loop/1(Iref) -> Current loop/1(Iref)
  Current Measurement1/1 -> Current loop1/2(imes), Current loop/2(imes)
  Pref/1 -> Divide/1
  Ves/1 -> Divide/2
  Divide/1 -> Current loop1/1(Iref)
  Current loop1/1(d) -> Manual Switch/1
  Manual Switch/1 -> Buck-Boost/1(d)
  Current loop/1(d) -> Manual Switch/2
  connections:
  Series RLC Branch1/RConn1 -- Current Measurement1/LConn1
  Buck-Boost/LConn1 -- Current Measurement1/RConn1
  Vout+/RConn1 -- Series RLC Branch/LConn1 -- Buck-Boost/RConn1
  Vout-/RConn1 -- Series RLC Branch/RConn1 -- Buck-Boost/RConn2
  Series RLC Branch1/LConn1 -- Vin+/RConn1
  Buck-Boost/LConn2 -- Vin-/RConn1

== system aconserversimulation/Diesel engine & control /Measurement of Generator ==
  m : Inport
  Bus Selector : BusSelector  OutputSignals=Stator current.is_a (pu),Stator current.is_b (pu),Stator current.is_c (pu)
  Bus Selector1 : BusSelector  OutputSignals="dq0 components.Stator voltage  vd (pu),dq0 components.Stator voltage  vq (pu),Mechanical.Rotor speed  wm  (pu),dq0 components.Stator voltage  vd (pu),dq0 components.Stator voltage  vq (pu),dq0 components.Field current  ifd (pu)"
  Mux : Mux  Inputs=2
  Mux1 : Mux  Inputs=2
  Scope2 : Scope  NumInputPorts=3
  wm : Outport  VectorParamsAs1DForOutWhenUnconnected=off
  vs_qd : Outport  Port=2  VectorParamsAs1DForOutWhenUnconnected=off
  is_qd : Outport  Port=3  VectorParamsAs1DForOutWhenUnconnected=off
  ifd : Outport  Port=4  VectorParamsAs1DForOutWhenUnconnected=off
  wires:
  Bus Selector1/1 -> Mux/1  "<Stator voltage  vd (pu)>"
  Bus Selector1/2 -> Mux/2  "<Stator voltage  vq (pu)>"
  Mux/1 -> vs_qd/1
  Bus Selector1/3 -> wm/1  "<Rotor speed  wm  (pu)>"
  Bus Selector1/4 -> Mux1/1  "<Stator voltage  vd (pu)>"
  Bus Selector1/5 -> Mux1/2  "<Stator voltage  vq (pu)>"
  Mux1/1 -> is_qd/1
  Bus Selector1/6 -> ifd/1  "<Field current  ifd (pu)>"
  Bus Selector/1 -> Scope2/1  "<is_a (pu)>"
  Bus Selector/2 -> Scope2/2  "<is_b (pu)>"
  m/1 -> Bus Selector/1, Bus Selector1/1
  Bus Selector/3 -> Scope2/3  "<is_c (pu)>"

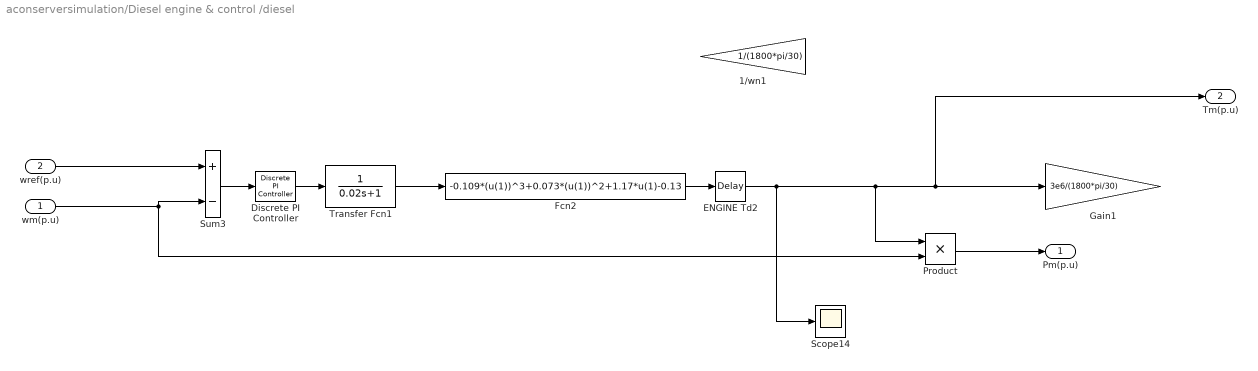
== system aconserversimulation/Diesel engine & control /diesel ==
  wm(p.u) : Inport
  wref(p.u) : Inport  Port=2
  1/wn1 : Gain  Gain=1/(1800*pi/30)
  Discrete PI Controller : powerlib_extras/Discrete  Control Blocks/Discrete PI Controller  Kp=8  Ki=4  Par_Limits=[3 -3]  Init=0  Ts=5e-6
      settings: SourceProductName=Simscape Electrical
  ENGINE Td2 : TransportDelay  DelayTime=0.023
  Fcn2 : Fcn  Expr=-0.109*(u(1))^3+0.073*(u(1))^2+1.17*u(1)-0.13
  Gain1 : Gain  Gain=3e6/(1800*pi/30)
  Product : Product  SaturateOnIntegerOverflow=on  InputSameDT=on  OutDataTypeStr=Inherit: Same as first input
  Scope14 : Scope
  Sum3 : Sum  Inputs=+-  SaturateOnIntegerOverflow=on  InputSameDT=on  OutDataTypeStr=Inherit: Same as first input
  Transfer Fcn1 : TransferFcn  Denominator=[0.02 1]
  Pm(p.u) : Outport  VectorParamsAs1DForOutWhenUnconnected=off
  Tm(p.u) : Outport  Port=2  VectorParamsAs1DForOutWhenUnconnected=off
  wires:
  wm(p.u)/1 -> Sum3/2, Product/2
  ENGINE Td2/1 -> Scope14/1, Product/1, Tm(p.u)/1, Gain1/1
  Discrete PI Controller/1 -> Transfer Fcn1/1
  Sum3/1 -> Discrete PI Controller/1
  Transfer Fcn1/1 -> Fcn2/1
  wref(p.u)/1 -> Sum3/1
  Fcn2/1 -> ENGINE Td2/1
  Product/1 -> Pm(p.u)/1

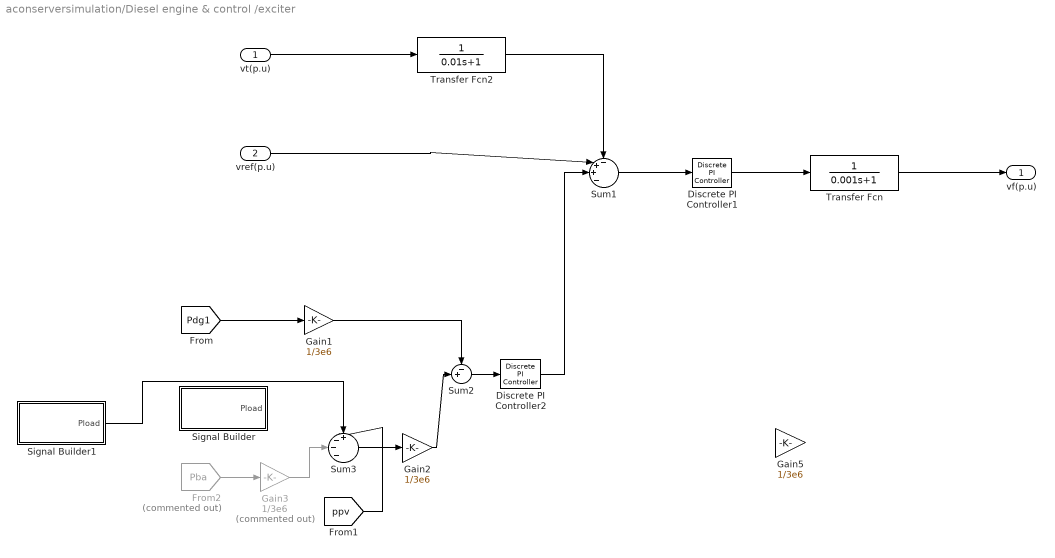
== system aconserversimulation/Diesel engine & control /exciter ==
  vt(p.u) : Inport
  vref(p.u) : Inport  Port=2
  Discrete PI Controller1 : powerlib_extras/Discrete  Control Blocks/Discrete PI Controller  Kp=30  Ki=10  Par_Limits=[10 -10]  Init=0  Ts=5e-6
      settings: SourceProductName=Simscape Electrical
  Discrete PI Controller2 : powerlib_extras/Discrete  Control Blocks/Discrete PI Controller  Kp=30  Ki=10  Par_Limits=[10 -10]  Init=0  Ts=5e-6
      settings: SourceProductName=Simscape Electrical
  From2 : From  Commented=on  GotoTag=Pba  TagVisibility=global
  Gain1 : Gain  Gain=1/3e6
  Gain2 : Gain  Gain=1/3e6
  Gain3 : Gain  Commented=on  Gain=1/3e6
  Gain5 : Gain  Gain=1/3e6
  Signal Builder : Subsystem  Tag=STV Subsys  LoadFcn=sigbuilder_block('load');  StartFcn=sigbuilder_block('start');  StopFcn=sigbuilder_block('stop');  ClipboardFcn=sigbuilder_block('clipboard');  mask(Sigbuilder block){tuvar=[0:10]}
      mask help: Simulink:masks:SigbuilderBlock_MD
      mask init:
      | if ~strcmp(get_param(bdroot(gcbh),'SimulationStatus'),'stopped') tuvar = sigbuilder_block('maskInit'); end
      settings: CopyFcn=sigbuilder_block('copy');  DeleteFcn=sigbuilder_block('delete');  ModelCloseFcn=sigbuilder_block('modelClose');  PreSaveFcn=sigbuilder_block('preSave');  PauseFcn=sigbuilder_block('pause');  ContinueFcn=sigbuilder_block('continue');  NameChangeFcn=sigbuilder_block('namechange');  OpenFcn=sigbuilder_block('open',[314.25 8.25 550.5 400.5 ]);  CloseFcn=sigbuilder_block('close');
      mask Display: plot(0, 0, 100, 100,[2, 2, 32, 32, 2], [68, 8, 8, 68, 68],[32, 2], [38, 38], [32, 19, 2],[53, 60, 44], [32, 17, 17, 2],[16, 16, 31, 31]);txt = getActiveGroup(gcbh);text(2, 100, txt,'verticalAlignment', 'top');
  Signal Builder1 : Subsystem  Tag=STV Subsys  LoadFcn=sigbuilder_block('load');  StartFcn=sigbuilder_block('start');  StopFcn=sigbuilder_block('stop');  ClipboardFcn=sigbuilder_block('clipboard');  mask(Sigbuilder block){tuvar=[0:10]}
      mask help: Simulink:masks:SigbuilderBlock_MD
      mask init:
      | if ~strcmp(get_param(bdroot(gcbh),'SimulationStatus'),'stopped') tuvar = sigbuilder_block('maskInit'); end
      settings: CopyFcn=sigbuilder_block('copy');  DeleteFcn=sigbuilder_block('delete');  ModelCloseFcn=sigbuilder_block('modelClose');  PreSaveFcn=sigbuilder_block('preSave');  PauseFcn=sigbuilder_block('pause');  ContinueFcn=sigbuilder_block('continue');  NameChangeFcn=sigbuilder_block('namechange');  OpenFcn=sigbuilder_block('open',[314.25 8.25 550.5 400.5 ]);  CloseFcn=sigbuilder_block('close');
      mask Display: plot(0, 0, 100, 100,[2, 2, 32, 32, 2], [68, 8, 8, 68, 68],[32, 2], [38, 38], [32, 19, 2],[53, 60, 44], [32, 17, 17, 2],[16, 16, 31, 31]);txt = getActiveGroup(gcbh);text(2, 100, txt,'verticalAlignment', 'top');
  Sum1 : Sum  Inputs=-++-|
  Sum2 : Sum  Inputs=-+|
  Sum3 : Sum  Inputs=+---|
  Transfer Fcn : TransferFcn  Denominator=[0.001 1]
  Transfer Fcn2 : TransferFcn  Denominator=[0.01 1]
  vf(p.u) : Outport  VectorParamsAs1DForOutWhenUnconnected=off
  wires:
  vt(p.u)/1 -> Transfer Fcn2/1
  Sum1/1 -> Discrete PI Controller1/1
  Discrete PI Controller1/1 -> Transfer Fcn/1
  Transfer Fcn/1 -> vf(p.u)/1
  vref(p.u)/1 -> Sum1/2
  Transfer Fcn2/1 -> Sum1/1
  Sum2/1 -> Discrete PI Controller2/1
  [Pdg1] -> Gain1/1
  Gain1/1 -> Sum2/1
  Discrete PI Controller2/1 -> Sum1/3
  From2/1 -> Gain3/1
  Gain3/1 -> Sum3/3
  Sum3/1 -> Gain2/1
  Gain2/1 -> Sum2/2
  Signal Builder1/1(Pload) -> Sum3/1
  [ppv] -> Sum3/2

== system aconserversimulation/Diesel engine & control 1/Measurement of Generator ==
  m : Inport
  Bus Selector1 : BusSelector  OutputSignals="dq0 components.Stator voltage  vd (pu),dq0 components.Stator voltage  vq (pu),Mechanical.Rotor speed  wm  (pu),dq0 components.Stator voltage  vd (pu),dq0 components.Stator voltage  vq (pu),dq0 components.Field current  ifd (pu)"
  Bus Selector3 : BusSelector  OutputSignals=Stator current.is_a (pu),Stator current.is_b (pu),Stator current.is_c (pu)
  Mux : Mux  Inputs=2
  Mux1 : Mux  Inputs=2
  Scope8 : Scope  NumInputPorts=3
  wm : Outport  VectorParamsAs1DForOutWhenUnconnected=off
  vs_qd : Outport  Port=2  VectorParamsAs1DForOutWhenUnconnected=off
  is_qd : Outport  Port=3  VectorParamsAs1DForOutWhenUnconnected=off
  ifd : Outport  Port=4  VectorParamsAs1DForOutWhenUnconnected=off
  wires:
  Bus Selector1/1 -> Mux/1  "<Stator voltage  vd (pu)>"
  Bus Selector1/2 -> Mux/2  "<Stator voltage  vq (pu)>"
  Mux/1 -> vs_qd/1
  Bus Selector1/3 -> wm/1  "<Rotor speed  wm  (pu)>"
  Bus Selector1/4 -> Mux1/1  "<Stator voltage  vd (pu)>"
  Bus Selector1/5 -> Mux1/2  "<Stator voltage  vq (pu)>"
  Mux1/1 -> is_qd/1
  Bus Selector1/6 -> ifd/1  "<Field current  ifd (pu)>"
  m/1 -> Bus Selector3/1, Bus Selector1/1
  Bus Selector3/2 -> Scope8/2  "<is_b (pu)>"
  Bus Selector3/1 -> Scope8/1  "<is_a (pu)>"
  Bus Selector3/3 -> Scope8/3  "<is_c (pu)>"

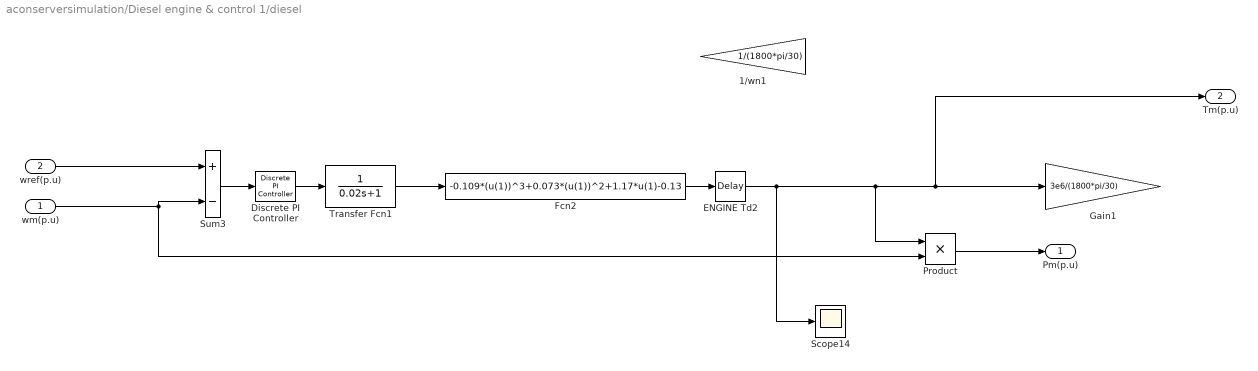
== system aconserversimulation/Diesel engine & control 1/diesel ==
  wm(p.u) : Inport
  wref(p.u) : Inport  Port=2
  1/wn1 : Gain  Gain=1/(1800*pi/30)
  Discrete PI Controller : powerlib_extras/Discrete  Control Blocks/Discrete PI Controller  Kp=8  Ki=4  Par_Limits=[3 -3]  Init=0  Ts=5e-6
      settings: SourceProductName=Simscape Electrical
  ENGINE Td2 : TransportDelay  DelayTime=0.023
  Fcn2 : Fcn  Expr=-0.109*(u(1))^3+0.073*(u(1))^2+1.17*u(1)-0.13
  Gain1 : Gain  Gain=3e6/(1800*pi/30)
  Product : Product  SaturateOnIntegerOverflow=on  InputSameDT=on  OutDataTypeStr=Inherit: Same as first input
  Scope14 : Scope
  Sum3 : Sum  Inputs=+-  SaturateOnIntegerOverflow=on  InputSameDT=on  OutDataTypeStr=Inherit: Same as first input
  Transfer Fcn1 : TransferFcn  Denominator=[0.02 1]
  Pm(p.u) : Outport  VectorParamsAs1DForOutWhenUnconnected=off
  Tm(p.u) : Outport  Port=2  VectorParamsAs1DForOutWhenUnconnected=off
  wires:
  wm(p.u)/1 -> Sum3/2, Product/2
  ENGINE Td2/1 -> Scope14/1, Product/1, Tm(p.u)/1, Gain1/1
  Discrete PI Controller/1 -> Transfer Fcn1/1
  Sum3/1 -> Discrete PI Controller/1
  Transfer Fcn1/1 -> Fcn2/1
  wref(p.u)/1 -> Sum3/1
  Fcn2/1 -> ENGINE Td2/1
  Product/1 -> Pm(p.u)/1
